simulink model "project1SimscapeForce"  (R2013a)
settings: Solver=ode3  StartTime=0.0  StopTime=30  FixedStep=.1  MaxStep=0.2  RelTol=1e-3
libraries: fl_lib x12, nesl_utility x6
settings Model: Creator=z  LastModifiedBy=z

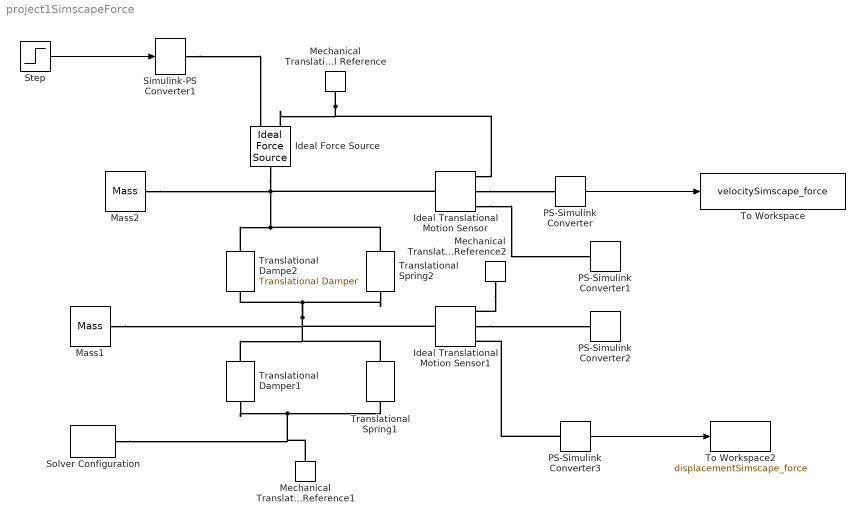
== system project1SimscapeForce ==
  Ideal Force Source : fl_lib/Mechanical/Mechanical Sources/Ideal Force Source  v_Log=off  f_Log=off  LocalVarNames=|v|f  LocalVarDescs=|v|f  LocalVarLogging=[0 0]
  Ideal Translational Motion Sensor : fl_lib/Mechanical/Mechanical Sensors/Ideal Translational Motion Sensor  offset=0 m  v_Log=off  f_Log=off  x_Log=off  LocalVarNames=|v|f|x  LocalVarDescs=|v|f|x  LocalVarLogging=[0 0 0]
  Ideal Translational Motion Sensor1 : fl_lib/Mechanical/Mechanical Sensors/Ideal Translational Motion Sensor  offset=0 m  v_Log=off  f_Log=off  x_Log=off  LocalVarNames=|v|f|x  LocalVarDescs=|v|f|x  LocalVarLogging=[0 0 0]
  "Mass1 " : fl_lib/Mechanical/Translational Elements/Mass  mass=2 kg  initial_velocity=0 m/s  f_Log=off  LocalVarNames=|f  LocalVarDescs=|f  LocalVarLogging=0
  Mass2 : fl_lib/Mechanical/Translational Elements/Mass  mass=1 kg  initial_velocity=0 m/s  f_Log=off  LocalVarNames=|f  LocalVarDescs=|f  LocalVarLogging=0
  Mechanical Translational Reference : fl_lib/Mechanical/Translational Elements/Mechanical Translational Reference  f_Log=off  LocalVarNames=|f  LocalVarDescs=|f  LocalVarLogging=0
  Mechanical Translational Reference1 : fl_lib/Mechanical/Translational Elements/Mechanical Translational Reference  f_Log=off  LocalVarNames=|f  LocalVarDescs=|f  LocalVarLogging=0
  Mechanical Translational Reference2 : fl_lib/Mechanical/Translational Elements/Mechanical Translational Reference  f_Log=off  LocalVarNames=|f  LocalVarDescs=|f  LocalVarLogging=0
  PS-Simulink Converter : nesl_utility/PS-Simulink Converter  PhysicalDomain=network_engine_domain  SubClassName=ps_output  LeftPortType=input  RightPortType=output  PseudoPeriodic=off  Frequencies=[]  Unit=m/s  AffineConversion=off
  PS-Simulink Converter1 : nesl_utility/PS-Simulink Converter  PhysicalDomain=network_engine_domain  SubClassName=ps_output  LeftPortType=input  RightPortType=output  PseudoPeriodic=off  Frequencies=[]  Unit=m  AffineConversion=off
  PS-Simulink Converter2 : nesl_utility/PS-Simulink Converter  PhysicalDomain=network_engine_domain  SubClassName=ps_output  LeftPortType=input  RightPortType=output  PseudoPeriodic=off  Frequencies=[]  Unit=m/s  AffineConversion=off
  PS-Simulink Converter3 : nesl_utility/PS-Simulink Converter  PhysicalDomain=network_engine_domain  SubClassName=ps_output  LeftPortType=input  RightPortType=output  PseudoPeriodic=off  Frequencies=[]  Unit=m  AffineConversion=off
  Simulink-PS Converter1 : nesl_utility/Simulink-PS Converter  PhysicalDomain=network_engine_domain  SubClassName=ps_input  LeftPortType=input  RightPortType=output  PseudoPeriodic=off  Frequencies=[]  NoiseDistribution=none  NoiseParameters=[]  Unit=1  AffineConversion=off  InputFiltering=off  SimscapeFilterOrder=1  InputFilterTimeConstant=0.001  UdotUserProvided=1
  Solver Configuration : nesl_utility/Solver Configuration  PhysicalDomain=network_engine_domain  SubClassName=solver  LeftPortType=input  RightPortType=generic  Accelerate=off  Tones=[]  Harmonics=[]  SimulateNoise=off  Profile=off  UseLocalSampling=off  EnableSwitchedLinearOptims=on  FrequencyDomain=off  UseCCode=off  UseNewInitialization=off  DoDC=off  ResidualTolerance=1e-09  UseLocalSolver=off  LocalSolverChoice=NE_BACKWARD_EULER_ADVANCER  LocalSolverSampleTime=0.001  DoFixedCost=off  MaxNonlinIter=3  MaxModeIter=2  LinearAlgebra=Sparse  DelaysMemoryBudget=1024
  Step : Step  Time=0  SampleTime=0
  To Workspace : ToWorkspace  VariableName=velocitySimscape_force  SampleTime=-1  SaveFormat=Timeseries
  To Workspace2 : ToWorkspace  VariableName=displacementSimscape_force  SampleTime=-1  SaveFormat=Timeseries
  Translational Dampe2 : fl_lib/Mechanical/Translational Elements/Translational Damper  D=2 N/(m/s)  f_Log=off  v_Log=off  LocalVarNames=|f|v  LocalVarDescs=|f|v  LocalVarLogging=[0 0]
  Translational Damper1 : fl_lib/Mechanical/Translational Elements/Translational Damper  D=1 N/(m/s)  f_Log=off  v_Log=off  LocalVarNames=|f|v  LocalVarDescs=|f|v  LocalVarLogging=[0 0]
  "Translational Spring1 " : fl_lib/Mechanical/Translational Elements/Translational Spring  spr_rate=2 N/m  init_def=0 m  f_Log=off  v_Log=off  x_Log=off  LocalVarNames=|f|v|x  LocalVarDescs=|f|v|x  LocalVarLogging=[0 0 0]
  Translational Spring2 : fl_lib/Mechanical/Translational Elements/Translational Spring  spr_rate=.2 N/m  init_def=0 m  f_Log=off  v_Log=off  x_Log=off  LocalVarNames=|f|v|x  LocalVarDescs=|f|v|x  LocalVarLogging=[0 0 0]
  wires:
  PS-Simulink Converter/1 -> To Workspace/1
  PS-Simulink Converter3/1 -> To Workspace2/1
  Step/1 -> Simulink-PS Converter1/1
  connections:
  Translational Spring2/RConn1 -- Ideal Translational Motion Sensor1/LConn1 -- Translational Damper1/LConn1 -- "Translational Spring1 "/LConn1 -- "Mass1 "/LConn1 -- Translational Dampe2/RConn1
  Mass2/LConn1 -- Ideal Force Source/LConn1 -- Translational Dampe2/LConn1 -- Translational Spring2/LConn1 -- Ideal Translational Motion Sensor/LConn1
  Mechanical Translational Reference/LConn1 -- Ideal Force Source/RConn2 -- Ideal Translational Motion Sensor/RConn1
  Simulink-PS Converter1/RConn1 -- Ideal Force Source/RConn1
  Ideal Translational Motion Sensor/RConn2 -- PS-Simulink Converter/LConn1
  Ideal Translational Motion Sensor/RConn3 -- PS-Simulink Converter1/LConn1
  Translational Damper1/RConn1 -- Mechanical Translational Reference1/LConn1 -- Solver Configuration/RConn1 -- "Translational Spring1 "/RConn1
  Mechanical Translational Reference2/LConn1 -- Ideal Translational Motion Sensor1/RConn1
  Ideal Translational Motion Sensor1/RConn2 -- PS-Simulink Converter2/LConn1
  PS-Simulink Converter3/LConn1 -- Ideal Translational Motion Sensor1/RConn3
